simulink model "eBike_simulink_arduinoMega"  (R2021b)
settings: Solver=ode3  StartTime=0.0  StopTime=inf  FixedStep=0.1  RelTol=1e-3  EnableMultiTasking=on
libraries: arduinolib x17, simulink x9, dspsigops x1
settings Model: FPTRunName=Active  ExtModeTrigDuration=2  Creator=HP  LastModifiedBy=adhip
settings SolverCC: AlgebraicLoopSolver=TrustRegion
settings DataIOCC: LimitDataPoints=on  SaveFormat=Array
settings OptimizationCC: ExpressionDepthLimit=2147483647  LifeSpan=Inf  MaxStackSize=64
settings DebuggingCC: MergeDetectMultiDrivingBlocksExec=none  FcnCallInpInsideContextMsg=warning  AllowSymbolicDim=off  StateNameClashWarn=warning  SFUnexpectedBacktrackingDiag=warning  SFNoUnconditionalDefaultTransitionDiag=warning  SFExecutionAtInitializationDiag=none  SFMachineParentedDataDiag=warning  ArithmeticOperatorsInVariantConditions=warning
settings HardwareCC: ProdBitPerInt=16  ProdBitPerPointer=16  ProdBitPerSizeT=16  ProdBitPerPtrDiffT=16  ProdLargestAtomicFloat=None  ProdWordSize=8  ProdHWDeviceType=Atmel->AVR  UseEmbeddedCoderFeatures=off  UseSimulinkCoderFeatures=off
settings ModelReferenceCC: PropagateSignalLabelsOutOfModel=off
settings SFSimCC: SimUseLocalCustomCode=off  CustomCodeUndefinedFunction=UseInterfaceOnly
settings RTWCC: Description=Embedded Coder  SystemTargetFile=ert.tlc  HardwareBoard=Arduino Mega 2560  TemplateMakefile=ert_default_tmf  GenerateReport=on  RTWVerbose=off  RTWUseLocalCustomCode=off  Toolchain=Arduino AVR  BuildConfiguration=Faster Runs  LaunchReport=on
settings CodeAppCC: ForceParamTrailComments=on  OperatorAnnotations=on  MangleLength=10  StateflowObjectComments=on  MATLABSourceComments=on
settings ERTTargetCC: MultiwordLength=2048  ERTCustomFileBanners=off  SupportContinuousTime=on  SupportNonInlinedSFcns=on  RemoveResetFunc=off  ModelStepFunctionPrototypeControlCompliant=off
settings ConfigComp: CovMetricSettings=dw  CovSaveCumulativeToWorkspaceVar=on  CovSaveSingleToWorkspaceVar=on  CovExternalEMLEnable=off  CovSFcnEnable=off

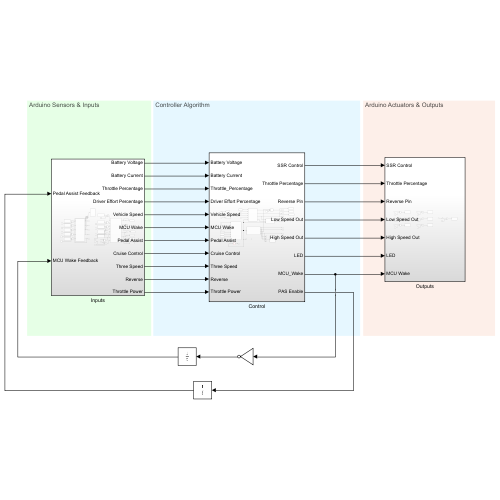
[thumbnail: Simulink's stored preview of the top-level diagram]
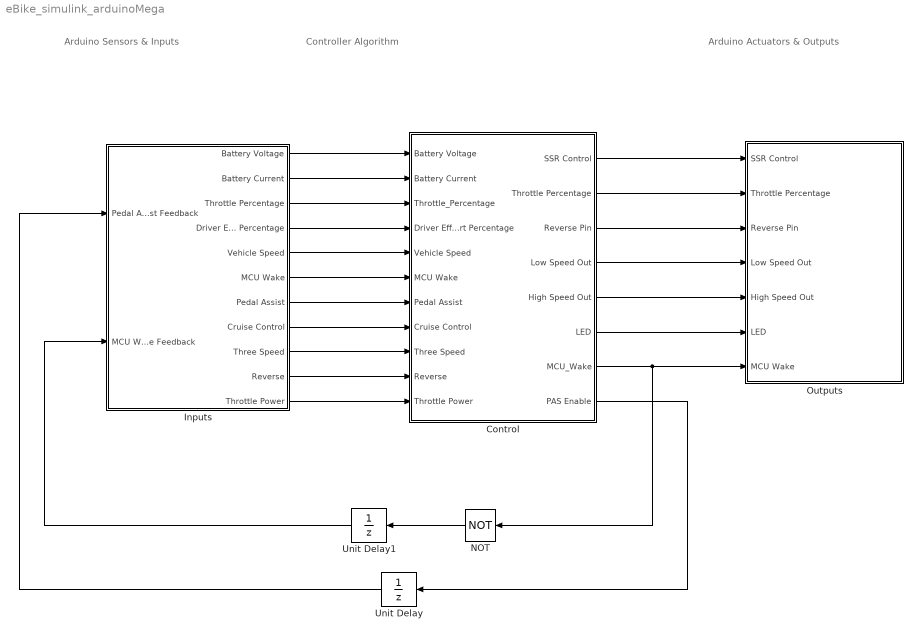
== system eBike_simulink_arduinoMega ==
  note: Arduino Actuators & Outputs
  note: Arduino Sensors & Inputs
  note: Controller Algorithm
  Control : Subsystem
  Inputs : Subsystem
  NOT : Logic  Operator=NOT  IconShape=distinctive  AllPortsSameDT=off  OutDataTypeStr=boolean
  Outputs : Subsystem
  Unit Delay : UnitDelay  SampleTime=-1  HasFrameUpgradeWarning=on
  Unit Delay1 : UnitDelay  SampleTime=-1  HasFrameUpgradeWarning=on
  wires:
  Inputs/1(Battery Voltage) -> Control/1(Battery Voltage)
  Inputs/2(Battery Current) -> Control/2(Battery Current)
  Inputs/3(Throttle Percentage) -> Control/3(Throttle_Percentage)
  Inputs/4(Driver Effort Percentage) -> Control/4(Driver Effort Percentage)
  Inputs/5(Vehicle Speed) -> Control/5(Vehicle Speed)
  Inputs/6(MCU Wake) -> Control/6(MCU Wake)
  Inputs/7(Pedal Assist) -> Control/7(Pedal Assist)
  Inputs/8(Cruise Control) -> Control/8(Cruise Control)
  Inputs/9(Three Speed) -> Control/9(Three Speed)
  Inputs/10(Reverse) -> Control/10(Reverse)
  Control/8(PAS Enable) -> Unit Delay/1
  Inputs/11(Throttle Power) -> Control/11(Throttle Power)
  Unit Delay/1 -> Inputs/1(Pedal Assist Feedback)
  Control/7(MCU_Wake) -> NOT/1, Outputs/7(MCU Wake)
  Unit Delay1/1 -> Inputs/2(MCU Wake Feedback)
  Control/1(SSR Control) -> Outputs/1(SSR Control)
  Control/3(Reverse Pin) -> Outputs/3(Reverse Pin)
  Control/4(Low Speed Out) -> Outputs/4(Low Speed Out)
  Control/5(High Speed Out) -> Outputs/5(High Speed Out)
  Control/6(LED) -> Outputs/6(LED)
  Control/2(Throttle Percentage) -> Outputs/2(Throttle Percentage)
  NOT/1 -> Unit Delay1/1

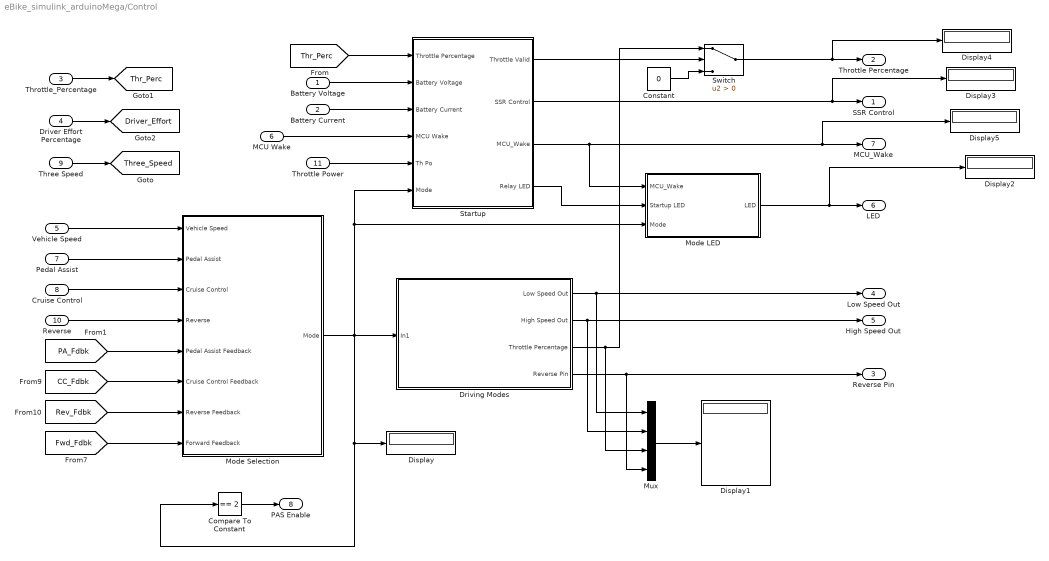
== system eBike_simulink_arduinoMega/Control ==
  Battery Voltage : Inport
  Battery Current : Inport  Port=2
  Throttle_Percentage : Inport  Port=3
  Driver Effort Percentage : Inport  Port=4
  Vehicle Speed : Inport  Port=5
  MCU Wake : Inport  Port=6
  Pedal Assist : Inport  Port=7
  Cruise Control : Inport  Port=8
  Three Speed : Inport  Port=9
  Reverse : Inport  Port=10
  Throttle Power : Inport  Port=11
  Compare To Constant : simulink/Logic and Bit Operations/Compare To Constant  relop===  const=2  OutDataTypeStr=boolean
  Constant : Constant  Value=0
  Display{,1..5} (6 alike) : Display
  Driving Modes : Subsystem
  Mode LED : Subsystem
  Mode Selection : Subsystem
  Mux : Mux
  Startup : Subsystem
  Switch : Switch  Criteria=u2 > Threshold
  SSR Control : Outport
  Throttle Percentage : Outport  Port=2
  Reverse Pin : Outport  Port=3
  Low Speed Out : Outport  Port=4
  High Speed Out : Outport  Port=5
  LED : Outport  Port=6
  MCU_Wake : Outport  Port=7
  PAS Enable : Outport  Port=8
  tag scope: Driver_Effort=global, Thr_Perc=global, Three_Speed=global
  wires:
  Pedal Assist/1 -> Mode Selection/2(Pedal Assist)
  Cruise Control/1 -> Mode Selection/3(Cruise Control)
  Reverse/1 -> Mode Selection/4(Reverse)
  Vehicle Speed/1 -> Mode Selection/1(Vehicle Speed)
  Three Speed/1 -> [Three_Speed]
  Throttle_Percentage/1 -> [Thr_Perc]
  Driver Effort Percentage/1 -> [Driver_Effort]
  [CC_Fdbk] -> Mode Selection/6(Cruise Control Feedback)
  [Fwd_Fdbk] -> Mode Selection/8(Forward Feedback)
  [Rev_Fdbk] -> Mode Selection/7(Reverse Feedback)
  Driving Modes/1(Low Speed Out) -> Mux/1, Low Speed Out/1
  Driving Modes/2(High Speed Out) -> Mux/2, High Speed Out/1
  Driving Modes/3(Throttle Percentage) -> Mux/3, Switch/1
  Driving Modes/4(Reverse Pin) -> Mux/4, Reverse Pin/1
  Battery Current/1 -> Startup/3(Battery Current)
  [Thr_Perc] -> Startup/1(Throttle Percentage)
  [PA_Fdbk] -> Mode Selection/5(Pedal Assist Feedback)
  Compare To Constant/1 -> PAS Enable/1
  Battery Voltage/1 -> Startup/2(Battery Voltage)
  Throttle Power/1 -> Startup/5(Th Po)
  Startup/4(Relay LED) -> Mode LED/2(Startup LED)
  Startup/3(MCU_Wake) -> Display5/1, MCU_Wake/1, Mode LED/1(MCU_Wake)
  Startup/1(Throttle Valid) -> Switch/2
  Constant/1 -> Switch/3
  Switch/1 -> Display4/1, Throttle Percentage/1
  Startup/2(SSR Control) -> Display3/1, SSR Control/1
  Mode LED/1(LED) -> Display2/1, LED/1
  Mode Selection/1(Mode) -> Display/1, Compare To Constant/1, Startup/6(Mode), Mode LED/3(Mode), Driving Modes/1(In1)
  Mux/1 -> Display1/1
  MCU Wake/1 -> Startup/4(MCU Wake)

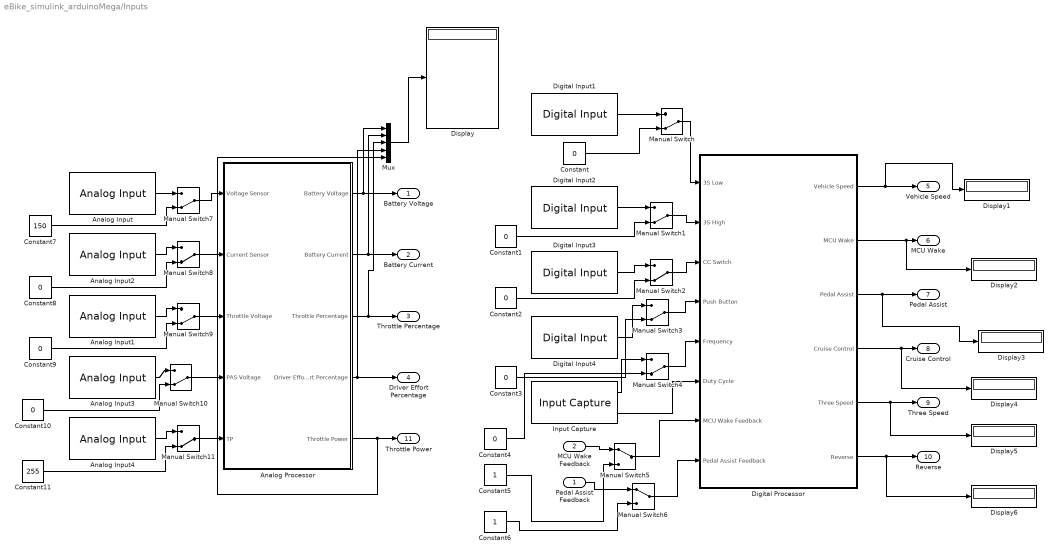
== system eBike_simulink_arduinoMega/Inputs ==
  Pedal Assist Feedback : Inport
  MCU Wake Feedback : Inport  Port=2
  Analog Input : arduinolib/Analog Input  pinNumber=15  ReadResultsOnly=off  ConversionTriggerSource=Software  ExternalTriggerType=uint32( 0 )  OutputDataType=uint16  EnableConversionCompleteNotify=off  EnableOuputStatus=off  SampleTime=-1  blockPlatform=arduino
  Analog Input1 : arduinolib/Analog Input  pinNumber=13  ReadResultsOnly=off  ConversionTriggerSource=Software  ExternalTriggerType=uint32( 0 )  OutputDataType=uint16  EnableConversionCompleteNotify=off  EnableOuputStatus=off  SampleTime=-1  blockPlatform=arduino
  Analog Input2 : arduinolib/Analog Input  pinNumber=14  ReadResultsOnly=off  ConversionTriggerSource=Software  ExternalTriggerType=uint32( 0 )  OutputDataType=uint16  EnableConversionCompleteNotify=off  EnableOuputStatus=off  SampleTime=-1  blockPlatform=arduino
  Analog Input3 : arduinolib/Analog Input  pinNumber=12  ReadResultsOnly=off  ConversionTriggerSource=Software  ExternalTriggerType=uint32( 0 )  OutputDataType=uint16  EnableConversionCompleteNotify=off  EnableOuputStatus=off  SampleTime=-1  blockPlatform=arduino
  Analog Input4 : arduinolib/Analog Input  pinNumber=11  ReadResultsOnly=off  ConversionTriggerSource=Software  ExternalTriggerType=uint32( 0 )  OutputDataType=uint16  EnableConversionCompleteNotify=off  EnableOuputStatus=off  SampleTime=-1  blockPlatform=arduino
  Analog Processor : Subsystem
  Constant{,1..4,8..10} (8 alike) : Constant  Value=0
  Constant11 : Constant  Value=255
  Constant5 : Constant
  Constant6 : Constant
  Constant7 : Constant  Value=150
  Digital Input1 : arduinolib/Digital Input  pinNumber=4  mode=Input Pullup  Direction=input  SampleTime=0.1  blockPlatform=arduino
  Digital Input2 : arduinolib/Digital Input  pinNumber=5  mode=Input Pullup  Direction=input  SampleTime=0.1  blockPlatform=arduino
  Digital Input3 : arduinolib/Digital Input  pinNumber=2  mode=Input Pullup  Direction=input  SampleTime=0.1  blockPlatform=arduino
  Digital Input4 : arduinolib/Digital Input  pinNumber=3  mode=Input Pullup  Direction=input  SampleTime=0.1  blockPlatform=arduino
  Digital Processor : Subsystem
  Display{,1..6} (7 alike) : Display
  Input Capture : arduinolib/Input Capture  InputCapturePinNumber=48  SampleTime=0.1
      settings: SourceProductBaseCode=ARDUINO
  Manual Switch{,1..4,7..11} (10 alike) : ManualSwitch  CurrentSetting=0
  Manual Switch5 : ManualSwitch
  Manual Switch6 : ManualSwitch
  Mux : Mux  Inputs=5
  Battery Voltage : Outport
  Battery Current : Outport  Port=2
  Throttle Percentage : Outport  Port=3
  Driver Effort Percentage : Outport  Port=4
  Vehicle Speed : Outport  Port=5
  MCU Wake : Outport  Port=6
  Pedal Assist : Outport  Port=7
  Cruise Control : Outport  Port=8
  Three Speed : Outport  Port=9
  Reverse : Outport  Port=10
  Throttle Power : Outport  Port=11
  wires:
  Manual Switch7/1 -> Analog Processor/1(Voltage Sensor)
  Manual Switch8/1 -> Analog Processor/2(Current Sensor)
  Manual Switch9/1 -> Analog Processor/3(Throttle Voltage)
  Manual Switch10/1 -> Analog Processor/4(PAS Voltage)
  Manual Switch/1 -> Digital Processor/1(3S Low)
  Manual Switch1/1 -> Digital Processor/2(3S High)
  Manual Switch2/1 -> Digital Processor/3(CC Switch)
  Manual Switch3/1 -> Digital Processor/4(Push Button)
  Manual Switch4/1 -> Digital Processor/5(Frequency)
  Input Capture/2 -> Digital Processor/6(Duty Cycle)
  Analog Processor/1(Battery Voltage) -> Mux/1, Battery Voltage/1
  Analog Processor/2(Battery Current) -> Mux/2, Battery Current/1
  Analog Processor/3(Throttle Percentage) -> Mux/3, Throttle Percentage/1
  Analog Processor/4(Driver Effort Percentage) -> Driver Effort Percentage/1, Mux/4
  Digital Processor/1(Vehicle Speed) -> Display1/1, Vehicle Speed/1
  Digital Processor/2(MCU Wake) -> Display2/1, MCU Wake/1
  Digital Processor/3(Pedal Assist) -> Display3/1, Pedal Assist/1
  Digital Processor/4(Cruise Control) -> Display4/1, Cruise Control/1
  Digital Processor/5(Three Speed) -> Display5/1, Three Speed/1
  Manual Switch6/1 -> Digital Processor/8(Pedal Assist Feedback)
  Manual Switch5/1 -> Digital Processor/7(MCU Wake Feedback)
  Analog Processor/5(Throttle Power) -> Mux/5, Throttle Power/1
  Manual Switch11/1 -> Analog Processor/5(TP)
  Digital Input1/1 -> Manual Switch/1
  Constant/1 -> Manual Switch/2
  Digital Input2/1 -> Manual Switch1/1
  Constant1/1 -> Manual Switch1/2
  Digital Input3/1 -> Manual Switch2/1
  Constant2/1 -> Manual Switch2/2
  Digital Input4/1 -> Manual Switch3/1
  Constant3/1 -> Manual Switch3/2
  Input Capture/1 -> Manual Switch4/1
  Constant4/1 -> Manual Switch4/2
  MCU Wake Feedback/1 -> Manual Switch5/1
  Constant5/1 -> Manual Switch5/2
  Pedal Assist Feedback/1 -> Manual Switch6/1
  Constant6/1 -> Manual Switch6/2
  Analog Input/1 -> Manual Switch7/1
  Constant7/1 -> Manual Switch7/2
  Analog Input2/1 -> Manual Switch8/1
  Constant8/1 -> Manual Switch8/2
  Analog Input1/1 -> Manual Switch9/1
  Constant9/1 -> Manual Switch9/2
  Analog Input3/1 -> Manual Switch10/1
  Constant10/1 -> Manual Switch10/2
  Analog Input4/1 -> Manual Switch11/1
  Constant11/1 -> Manual Switch11/2
  Mux/1 -> Display/1
  Digital Processor/6(Reverse) -> Display6/1, Reverse/1

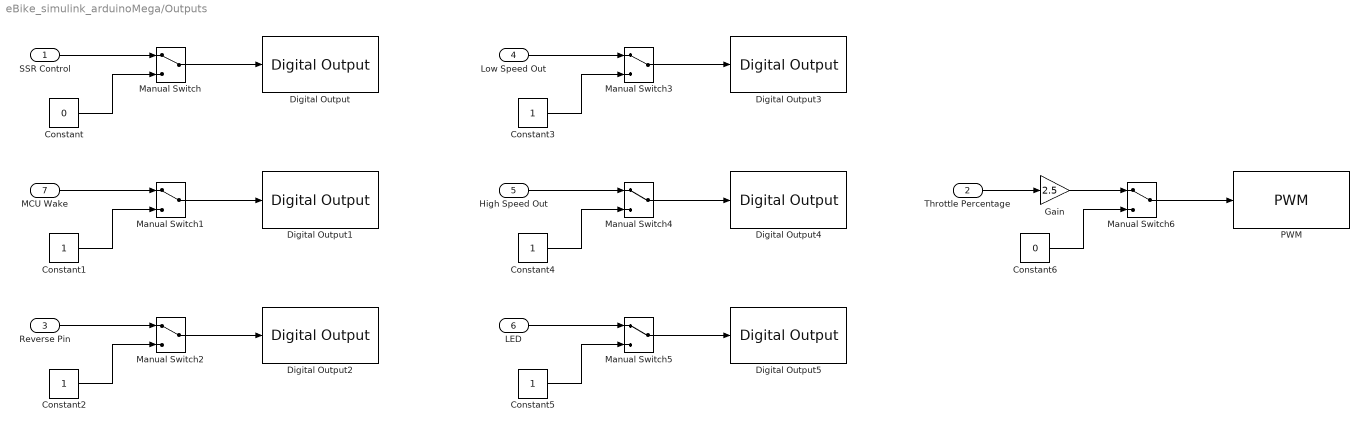
== system eBike_simulink_arduinoMega/Outputs ==
  SSR Control : Inport
  Throttle Percentage : Inport  Port=2
  Reverse Pin : Inport  Port=3
  Low Speed Out : Inport  Port=4
  High Speed Out : Inport  Port=5
  LED : Inport  Port=6
  MCU Wake : Inport  Port=7
  Constant : Constant  Value=0
  Constant{1..5} (5 alike) : Constant
  Constant6 : Constant  Value=0
  Digital Output : arduinolib/Digital Output  pinNumber=9  Direction=output  blockPlatform=arduino
  Digital Output1 : arduinolib/Digital Output  pinNumber=10  Direction=output  blockPlatform=arduino
  Digital Output2 : arduinolib/Digital Output  pinNumber=6  Direction=output  blockPlatform=arduino
  Digital Output3 : arduinolib/Digital Output  pinNumber=8  Direction=output  blockPlatform=arduino
  Digital Output4 : arduinolib/Digital Output  pinNumber=7  Direction=output  blockPlatform=arduino
  Digital Output5 : arduinolib/Digital Output  pinNumber=11  Direction=output  blockPlatform=arduino
  Gain : Gain  Gain=2.5
  Manual Switch{,1..6} (7 alike) : ManualSwitch
  PWM : arduinolib/PWM  pinNumber=12  frequencyType=Default  desiredFrequency=490.2  achievableFrequency=490.2
  wires:
  Manual Switch/1 -> Digital Output/1
  Constant/1 -> Manual Switch/2
  SSR Control/1 -> Manual Switch/1
  MCU Wake/1 -> Manual Switch1/1
  Constant1/1 -> Manual Switch1/2
  Manual Switch1/1 -> Digital Output1/1
  Manual Switch2/1 -> Digital Output2/1
  Constant2/1 -> Manual Switch2/2
  Reverse Pin/1 -> Manual Switch2/1
  LED/1 -> Manual Switch5/1
  Constant5/1 -> Manual Switch5/2
  Manual Switch5/1 -> Digital Output5/1
  Manual Switch4/1 -> Digital Output4/1
  Constant4/1 -> Manual Switch4/2
  High Speed Out/1 -> Manual Switch4/1
  Low Speed Out/1 -> Manual Switch3/1
  Constant3/1 -> Manual Switch3/2
  Manual Switch3/1 -> Digital Output3/1
  Manual Switch6/1 -> PWM/1
  Constant6/1 -> Manual Switch6/2
  Throttle Percentage/1 -> Gain/1
  Gain/1 -> Manual Switch6/1

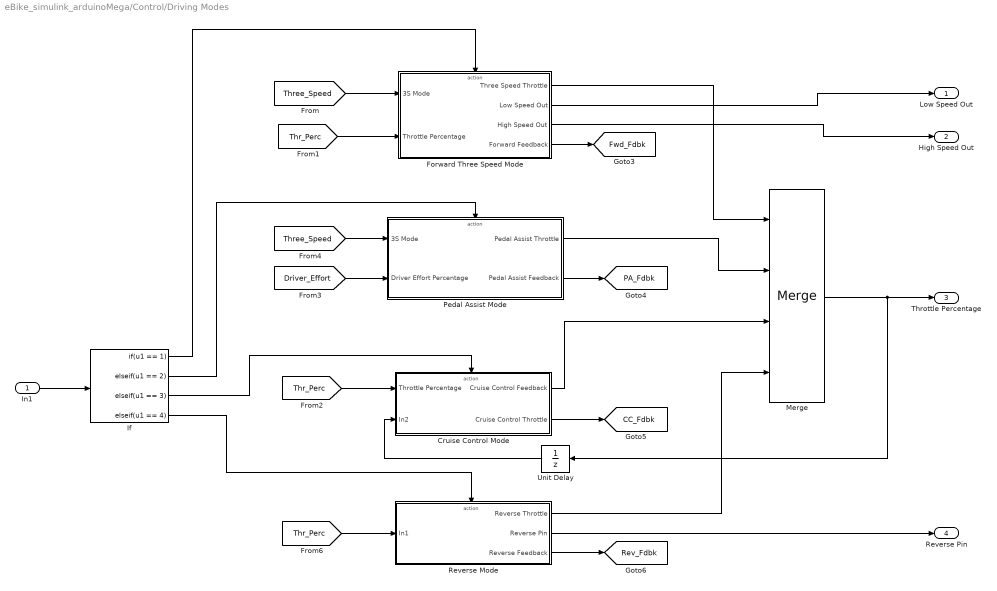
== system eBike_simulink_arduinoMega/Control/Driving Modes ==
  In1 : Inport
  Cruise Control Mode : Subsystem  TreatAsAtomicUnit=on
  Forward Three Speed Mode : Subsystem  TreatAsAtomicUnit=on
  If : If  IfExpression=u1 == 1  ElseIfExpressions=u1 == 2,u1 == 3,u1 == 4  ShowElse=off
  Merge : Merge  Inputs=4
  Pedal Assist Mode : Subsystem  TreatAsAtomicUnit=on
  Reverse Mode : Subsystem  TreatAsAtomicUnit=on
  Unit Delay : UnitDelay  SampleTime=-1  HasFrameUpgradeWarning=on
  Low Speed Out : Outport
  High Speed Out : Outport  Port=2
  Throttle Percentage : Outport  Port=3
  Reverse Pin : Outport  Port=4
  tag scope: CC_Fdbk=global, Fwd_Fdbk=global, PA_Fdbk=global, Rev_Fdbk=global
  wires:
  [Thr_Perc] -> Cruise Control Mode/1(Throttle Percentage)
  Reverse Mode/1(Reverse Throttle) -> Merge/4
  Cruise Control Mode/1(Cruise Control Feedback) -> Merge/3
  If/4 -> Reverse Mode/Action
  Reverse Mode/2(Reverse Pin) -> Reverse Pin/1
  [Thr_Perc] -> Reverse Mode/1(In1)
  Forward Three Speed Mode/1(Three Speed Throttle) -> Merge/1
  Pedal Assist Mode/1(Pedal Assist Throttle) -> Merge/2
  [Three_Speed] -> Forward Three Speed Mode/1(3S Mode)
  If/2 -> Pedal Assist Mode/Action
  If/3 -> Cruise Control Mode/Action
  Forward Three Speed Mode/3(High Speed Out) -> High Speed Out/1
  Reverse Mode/3(Reverse Feedback) -> [Rev_Fdbk]
  Forward Three Speed Mode/2(Low Speed Out) -> Low Speed Out/1
  If/1 -> Forward Three Speed Mode/Action
  In1/1 -> If/1
  Forward Three Speed Mode/4(Forward Feedback) -> [Fwd_Fdbk]
  [Driver_Effort] -> Pedal Assist Mode/2(Driver Effort Percentage)
  [Thr_Perc] -> Forward Three Speed Mode/2(Throttle Percentage)
  Cruise Control Mode/2(Cruise Control Throttle) -> [CC_Fdbk]
  [Three_Speed] -> Pedal Assist Mode/1(3S Mode)
  Pedal Assist Mode/2(Pedal Assist Feedback) -> [PA_Fdbk]
  Merge/1 -> Unit Delay/1, Throttle Percentage/1
  Unit Delay/1 -> Cruise Control Mode/2(In2)

== system eBike_simulink_arduinoMega/Control/Mode LED ==
  MCU_Wake : Inport
  Startup LED : Inport  Port=2
  Mode : Inport  Port=3
  Chart : Stateflow chart  TreatAsAtomicUnit=on
  Compare To Constant : simulink/Logic and Bit Operations/Compare To Constant  relop===  const=3.0  OutDataTypeStr=boolean
  Compare To Constant1 : simulink/Logic and Bit Operations/Compare To Constant  relop===  const=4  OutDataTypeStr=boolean
  Compare To Constant2 : simulink/Logic and Bit Operations/Compare To Constant  relop===  const=2  OutDataTypeStr=boolean
  Data Type Conversion : DataTypeConversion  OutDataTypeStr=boolean
  LED : Outport
  wires:
  Startup LED/1 -> Data Type Conversion/1
  Mode/1 -> Compare To Constant2/1, Compare To Constant1/1, Compare To Constant/1
  Compare To Constant/1 -> Chart/3(CC_LED)
  Compare To Constant1/1 -> Chart/4(Rev_LED)
  Compare To Constant2/1 -> Chart/5(PA_LED)
  MCU_Wake/1 -> Chart/1(MCU_Wake)
  Chart/1(relay_LED) -> LED/1
  Data Type Conversion/1 -> Chart/2(Startup_LED)

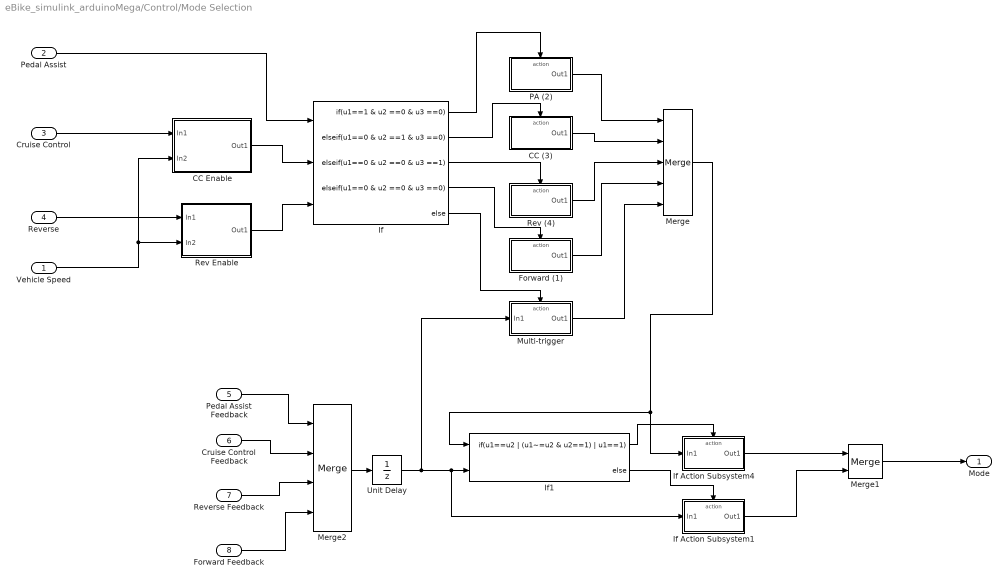
== system eBike_simulink_arduinoMega/Control/Mode Selection ==
  Vehicle Speed : Inport
  Pedal Assist : Inport  Port=2
  Cruise Control : Inport  Port=3
  Reverse : Inport  Port=4
  Pedal Assist Feedback : Inport  Port=5
  Cruise Control Feedback : Inport  Port=6
  Reverse Feedback : Inport  Port=7
  Forward Feedback : Inport  Port=8
  CC (3) : Subsystem  TreatAsAtomicUnit=on
  CC Enable : Subsystem
  Forward (1) : Subsystem  TreatAsAtomicUnit=on
  If : If  NumInputs=3  IfExpression=u1==1 & u2 ==0 & u3 ==0  ElseIfExpressions=u1==0 & u2 ==1 & u3 ==0,u1==0 & u2 ==0 & u3 ==1,u1==0 & u2 ==0 & u3 ==0
  If Action Subsystem1 : Subsystem  TreatAsAtomicUnit=on
  If Action Subsystem4 : Subsystem  TreatAsAtomicUnit=on
  If1 : If  NumInputs=2  IfExpression=u1==u2 | (u1~=u2 & u2==1) | u1==1
  Merge : Merge  Inputs=5
  Merge1 : Merge
  Merge2 : Merge  Inputs=4
  Multi-trigger : Subsystem  TreatAsAtomicUnit=on
  PA (2) : Subsystem  TreatAsAtomicUnit=on
  Rev (4) : Subsystem  TreatAsAtomicUnit=on
  Rev Enable : Subsystem
  Unit Delay : UnitDelay  InitialCondition=1  SampleTime=-1  HasFrameUpgradeWarning=on
  Mode : Outport
  wires:
  Pedal Assist/1 -> If/1
  If/1 -> PA (2)/Action
  If/2 -> CC (3)/Action
  If/3 -> Rev (4)/Action
  PA (2)/1(Out1) -> Merge/1
  CC (3)/1(Out1) -> Merge/2
  Rev (4)/1(Out1) -> Merge/3
  Forward (1)/1(Out1) -> Merge/4
  Pedal Assist Feedback/1 -> Merge2/1
  Cruise Control Feedback/1 -> Merge2/2
  Reverse Feedback/1 -> Merge2/3
  Forward Feedback/1 -> Merge2/4
  Merge2/1 -> Unit Delay/1
  Merge/1 -> If1/1, If Action Subsystem4/1(In1)
  If1/1 -> If Action Subsystem4/Action
  If Action Subsystem4/1(Out1) -> Merge1/1
  Merge1/1 -> Mode/1
  Vehicle Speed/1 -> Rev Enable/2(In2), CC Enable/2(In2)
  If1/2 -> If Action Subsystem1/Action
  If Action Subsystem1/1(Out1) -> Merge1/2
  If/4 -> Forward (1)/Action
  If/5 -> Multi-trigger/Action
  Reverse/1 -> Rev Enable/1(In1)
  Rev Enable/1(Out1) -> If/3
  Cruise Control/1 -> CC Enable/1(In1)
  CC Enable/1(Out1) -> If/2
  Multi-trigger/1(Out1) -> Merge/5
  Unit Delay/1 -> Multi-trigger/1(In1), If Action Subsystem1/1(In1), If1/2

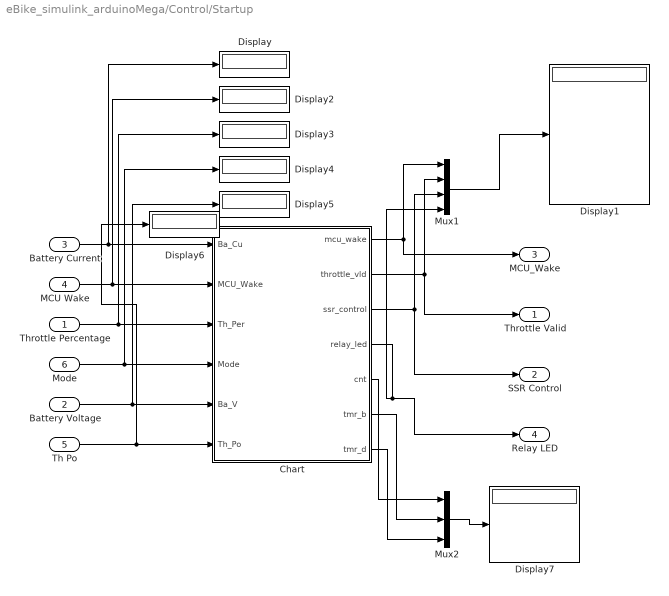
== system eBike_simulink_arduinoMega/Control/Startup ==
  Throttle Percentage : Inport
  Battery Voltage : Inport  Port=2
  Battery Current : Inport  Port=3
  MCU Wake : Inport  Port=4
  Th Po : Inport  Port=5
  Mode : Inport  Port=6
  Chart : Stateflow chart  TreatAsAtomicUnit=on
  Display{,1..7} (8 alike) : Display
  Mux1 : Mux
  Mux2 : Mux  Inputs=3
  Throttle Valid : Outport
  SSR Control : Outport  Port=2
  MCU_Wake : Outport  Port=3
  Relay LED : Outport  Port=4
  wires:
  MCU Wake/1 -> Display2/1, Chart/2(MCU_Wake)
  Throttle Percentage/1 -> Display3/1, Chart/3(Th_Per)
  Mode/1 -> Display4/1, Chart/4(Mode)
  Battery Voltage/1 -> Display5/1, Chart/5(Ba_V)
  Th Po/1 -> Display6/1, Chart/6(Th_Po)
  Chart/1(mcu_wake) -> MCU_Wake/1, Mux1/1
  Chart/2(throttle_vld) -> Throttle Valid/1, Mux1/2
  Chart/3(ssr_control) -> SSR Control/1, Mux1/3
  Chart/4(relay_led) -> Relay LED/1, Mux1/4
  Battery Current/1 -> Display/1, Chart/1(Ba_Cu)
  Mux1/1 -> Display1/1
  Chart/5(cnt) -> Mux2/1
  Chart/6(tmr_b) -> Mux2/2
  Chart/7(tmr_d) -> Mux2/3
  Mux2/1 -> Display7/1

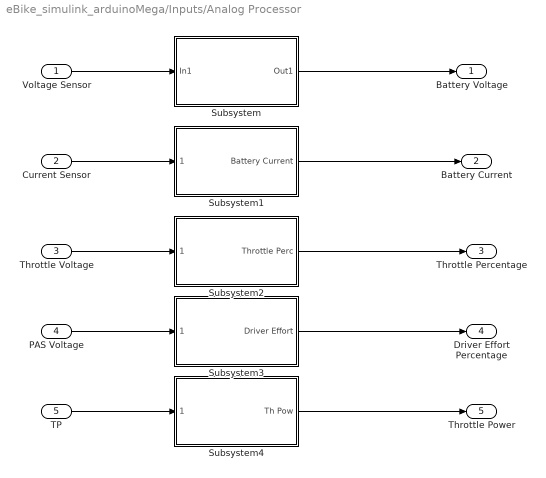
== system eBike_simulink_arduinoMega/Inputs/Analog Processor ==
  Voltage Sensor : Inport
  Current Sensor : Inport  Port=2
  Throttle Voltage : Inport  Port=3
  PAS Voltage : Inport  Port=4
  TP : Inport  Port=5
  Subsystem : Subsystem
  Subsystem1 : Subsystem
  Subsystem2 : Subsystem
  Subsystem3 : Subsystem
  Subsystem4 : Subsystem
  Battery Voltage : Outport
  Battery Current : Outport  Port=2
  Throttle Percentage : Outport  Port=3
  Driver Effort Percentage : Outport  Port=4
  Throttle Power : Outport  Port=5
  wires:
  Voltage Sensor/1 -> Subsystem/1(In1)
  Subsystem/1(Out1) -> Battery Voltage/1
  Current Sensor/1 -> Subsystem1/1(1)
  Subsystem1/1(Battery Current) -> Battery Current/1
  Throttle Voltage/1 -> Subsystem2/1(1)
  Subsystem2/1(Throttle Perc) -> Throttle Percentage/1
  PAS Voltage/1 -> Subsystem3/1(1)
  Subsystem3/1(Driver Effort) -> Driver Effort Percentage/1
  TP/1 -> Subsystem4/1(1)
  Subsystem4/1(Th Pow) -> Throttle Power/1

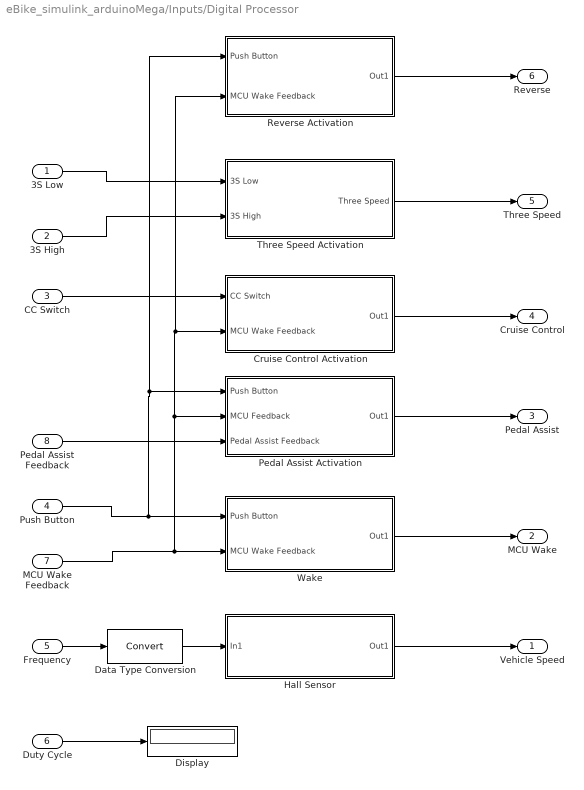
== system eBike_simulink_arduinoMega/Inputs/Digital Processor ==
  3S Low : Inport
  3S High : Inport  Port=2
  CC Switch : Inport  Port=3
  Push Button : Inport  Port=4
  Frequency : Inport  Port=5
  Duty Cycle : Inport  Port=6
  MCU Wake Feedback : Inport  Port=7
  Pedal Assist Feedback : Inport  Port=8
  Cruise Control Activation : Subsystem
  Data Type Conversion : DataTypeConversion
  Display : Display
  Hall Sensor : Subsystem
  Pedal Assist Activation : Subsystem
  Reverse Activation : Subsystem
  Three Speed Activation : Subsystem
  Wake : Subsystem
  Vehicle Speed : Outport
  MCU Wake : Outport  Port=2
  Pedal Assist : Outport  Port=3
  Cruise Control : Outport  Port=4
  Three Speed : Outport  Port=5
  Reverse : Outport  Port=6
  wires:
  Duty Cycle/1 -> Display/1
  Push Button/1 -> Reverse Activation/1(Push Button), Pedal Assist Activation/1(Push Button), Wake/1(Push Button)
  MCU Wake Feedback/1 -> Reverse Activation/2(MCU Wake Feedback), Cruise Control Activation/2(MCU Wake Feedback), Pedal Assist Activation/2(MCU Feedback), Wake/2(MCU Wake Feedback)
  Wake/1(Out1) -> MCU Wake/1
  Pedal Assist Activation/1(Out1) -> Pedal Assist/1
  CC Switch/1 -> Cruise Control Activation/1(CC Switch)
  Cruise Control Activation/1(Out1) -> Cruise Control/1
  3S Low/1 -> Three Speed Activation/1(3S Low)
  3S High/1 -> Three Speed Activation/2(3S High)
  Reverse Activation/1(Out1) -> Reverse/1
  Frequency/1 -> Data Type Conversion/1
  Hall Sensor/1(Out1) -> Vehicle Speed/1
  Three Speed Activation/1(Three Speed) -> Three Speed/1
  Pedal Assist Feedback/1 -> Pedal Assist Activation/3(Pedal Assist Feedback)
  Data Type Conversion/1 -> Hall Sensor/1(In1)

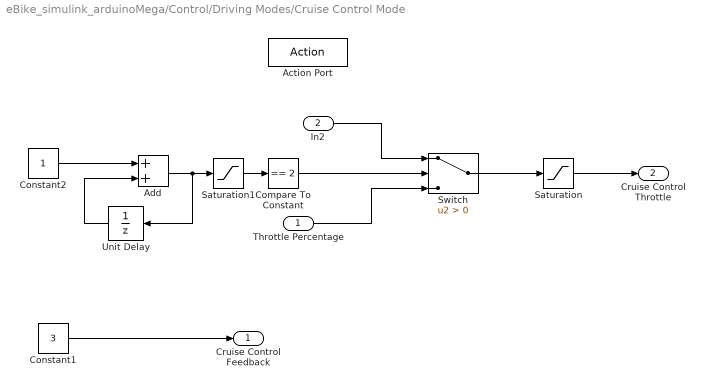
== system eBike_simulink_arduinoMega/Control/Driving Modes/Cruise Control Mode ==
  Throttle Percentage : Inport
  In2 : Inport  Port=2
  Action Port : ActionPort  InitializeStates=reset  ActionPortLabel=elseif(u1 == 3)
  Add : Sum
  Compare To Constant : simulink/Logic and Bit Operations/Compare To Constant  relop===  const=2  OutDataTypeStr=boolean
  Constant1 : Constant  Value=3
  Constant2 : Constant
  Saturation : Saturate  UpperLimit=50  LowerLimit=20
  Saturation1 : Saturate  UpperLimit=2  LowerLimit=0
  Switch : Switch  Criteria=u2 > Threshold
  Unit Delay : UnitDelay  SampleTime=-1  HasFrameUpgradeWarning=on
  Cruise Control Feedback : Outport
  Cruise Control Throttle : Outport  Port=2
  wires:
  In2/1 -> Switch/1
  Throttle Percentage/1 -> Switch/3
  Unit Delay/1 -> Add/2
  Saturation/1 -> Cruise Control Throttle/1
  Compare To Constant/1 -> Switch/2
  Constant1/1 -> Cruise Control Feedback/1
  Saturation1/1 -> Compare To Constant/1
  Add/1 -> Saturation1/1, Unit Delay/1
  Constant2/1 -> Add/1
  Switch/1 -> Saturation/1

== system eBike_simulink_arduinoMega/Control/Driving Modes/Forward Three Speed Mode ==
  3S Mode : Inport
  Throttle Percentage : Inport  Port=2
  Action Port : ActionPort  InitializeStates=reset  ActionPortLabel=if(u1 == 1)
  Constant : Constant
  High Speed Mapping : Subsystem  TreatAsAtomicUnit=on
  If : If  IfExpression=u1 == 1  ElseIfExpressions=u1 == 3
  Linear Mapping : Subsystem  TreatAsAtomicUnit=on
  Low Speed Mapping : Subsystem  TreatAsAtomicUnit=on
  Merge : Merge  Inputs=3
  Three Speed Throttle : Outport
  Low Speed Out : Outport  Port=2
  High Speed Out : Outport  Port=3
  Forward Feedback : Outport  Port=4  InitialOutput=1
  wires:
  3S Mode/1 -> If/1
  If/1 -> Low Speed Mapping/Action
  Throttle Percentage/1 -> Low Speed Mapping/1(Throttle Percentage), Linear Mapping/1(Throttle Percentage), High Speed Mapping/1(Throttle Percentage)
  Low Speed Mapping/1(Out1) -> Merge/1
  Linear Mapping/1(Out1) -> Merge/2
  High Speed Mapping/1(Out1) -> Merge/3
  Merge/1 -> Three Speed Throttle/1
  Low Speed Mapping/2(Low Speed Out) -> Low Speed Out/1
  High Speed Mapping/2(High Speed Out) -> High Speed Out/1
  Constant/1 -> Forward Feedback/1
  If/2 -> High Speed Mapping/Action
  If/3 -> Linear Mapping/Action

== system eBike_simulink_arduinoMega/Control/Driving Modes/Pedal Assist Mode ==
  3S Mode : Inport
  Driver Effort Percentage : Inport  Port=2
  Action Port : ActionPort  InitializeStates=reset  ActionPortLabel=elseif(u1 == 2)
  Constant : Constant  Value=2
  If : If  IfExpression=u1 == 1  ElseIfExpressions=u1 == 2,u1 == 3  ShowElse=off
  Level 1 : Subsystem  TreatAsAtomicUnit=on
  Level 2 : Subsystem  TreatAsAtomicUnit=on
  Level 3 : Subsystem  TreatAsAtomicUnit=on
  Merge : Merge  Inputs=3
  Pedal Assist Throttle : Outport
  Pedal Assist Feedback : Outport  Port=2
  wires:
  Constant/1 -> Pedal Assist Feedback/1
  Merge/1 -> Pedal Assist Throttle/1
  Level 3/1(L3 Throttle) -> Merge/3
  Level 2/1(L2 Throttle) -> Merge/2
  Level 1/1(L1 Throttle) -> Merge/1
  Driver Effort Percentage/1 -> Level 3/1(Driver Effort), Level 1/1(Driver Effort), Level 2/1(Driver Effort)
  If/3 -> Level 3/Action
  If/2 -> Level 2/Action
  If/1 -> Level 1/Action
  3S Mode/1 -> If/1

== system eBike_simulink_arduinoMega/Control/Driving Modes/Reverse Mode ==
  In1 : Inport
  Action Port : ActionPort  InitializeStates=reset  ActionPortLabel=elseif(u1 == 4)
  Constant1 : Constant
  Constant2 : Constant  Value=4
  Reverse Throttle : Outport
  Reverse Pin : Outport  Port=2  OutputWhenDisabled=reset  InitialOutput=0
  Reverse Feedback : Outport  Port=3
  wires:
  In1/1 -> Reverse Throttle/1
  Constant1/1 -> Reverse Pin/1
  Constant2/1 -> Reverse Feedback/1

== system eBike_simulink_arduinoMega/Control/Mode Selection/CC (3) ==
  Action Port : ActionPort  ActionPortLabel=elseif(u1==0 & u2 ==1 & u3 ==0)
  Constant : Constant  Value=3
  Out1 : Outport
  wires:
  Constant/1 -> Out1/1

== system eBike_simulink_arduinoMega/Control/Mode Selection/CC Enable ==
  In1 : Inport
  In2 : Inport  Port=2
  AND1 : Logic  IconShape=distinctive  AllPortsSameDT=off  OutDataTypeStr=boolean
  Constant1 : Constant  Value=10
  Less Than1 : RelationalOperator  Operator=<  OutDataTypeStr=boolean  RndMeth=Simplest
  Out1 : Outport
  wires:
  Constant1/1 -> Less Than1/2
  In1/1 -> AND1/1
  In2/1 -> Less Than1/1
  Less Than1/1 -> AND1/2
  AND1/1 -> Out1/1

== system eBike_simulink_arduinoMega/Control/Mode Selection/Forward (1) ==
  Action Port : ActionPort  ActionPortLabel=elseif(u1==0 & u2 ==0 & u3 ==0)
  Constant : Constant
  Out1 : Outport
  wires:
  Constant/1 -> Out1/1

== system eBike_simulink_arduinoMega/Control/Mode Selection/If Action Subsystem1 ==
  In1 : Inport
  Action Port : ActionPort  ActionPortLabel=else
  Out1 : Outport
  wires:
  In1/1 -> Out1/1

== system eBike_simulink_arduinoMega/Control/Mode Selection/If Action Subsystem4 ==
  In1 : Inport
  Action Port : ActionPort  ActionPortLabel=if(u1==u2 | (u1~=u2 & u2==1) | u1==1)
  Out1 : Outport
  wires:
  In1/1 -> Out1/1

== system eBike_simulink_arduinoMega/Control/Mode Selection/Multi-trigger ==
  In1 : Inport
  Action Port : ActionPort  ActionPortLabel=else
  Out1 : Outport
  wires:
  In1/1 -> Out1/1

== system eBike_simulink_arduinoMega/Control/Mode Selection/PA (2) ==
  Action Port : ActionPort  ActionPortLabel=if(u1==1 & u2 ==0 & u3 ==0)
  Constant : Constant  Value=2
  Out1 : Outport
  wires:
  Constant/1 -> Out1/1

== system eBike_simulink_arduinoMega/Control/Mode Selection/Rev (4) ==
  Action Port : ActionPort  ActionPortLabel=elseif(u1==0 & u2 ==0 & u3 ==1)
  Constant : Constant  Value=4
  Out1 : Outport
  wires:
  Constant/1 -> Out1/1

== system eBike_simulink_arduinoMega/Control/Mode Selection/Rev Enable ==
  In1 : Inport
  In2 : Inport  Port=2
  AND : Logic  IconShape=distinctive  AllPortsSameDT=off  OutDataTypeStr=boolean
  Constant : Constant
  Less Than : RelationalOperator  Operator=<  OutDataTypeStr=boolean  RndMeth=Simplest
  Out1 : Outport
  wires:
  AND/1 -> Out1/1
  In2/1 -> Less Than/1
  Constant/1 -> Less Than/2
  Less Than/1 -> AND/2
  In1/1 -> AND/1

== system eBike_simulink_arduinoMega/Inputs/Analog Processor/Subsystem ==
  In1 : Inport
  Add : Sum  Inputs=+-
  Add1 : Sum  Inputs=+-
  Divide : Product  Inputs=/*
  Gain : Gain  Gain=40
  High ADC Voltage Count : Constant  Value=255
  Low ADC Voltage Count : Constant  Value=0
  Out1 : Outport
  wires:
  In1/1 -> Add/1
  Low ADC Voltage Count/1 -> Add1/2, Add/2
  High ADC Voltage Count/1 -> Add1/1
  Add/1 -> Divide/2
  Add1/1 -> Divide/1
  Divide/1 -> Gain/1
  Gain/1 -> Out1/1

== system eBike_simulink_arduinoMega/Inputs/Analog Processor/Subsystem1 ==
  1 : Inport
  Add : Sum  Inputs=+-
  Add1 : Sum  Inputs=+-
  Divide : Product  Inputs=/*
  Gain : Gain  Gain=20
  High ADC Voltage Count : Constant  Value=255
  Low ADC Voltage Count : Constant  Value=0
  Battery Current : Outport
  wires:
  Gain/1 -> Battery Current/1
  Divide/1 -> Gain/1
  Add1/1 -> Divide/1
  Add/1 -> Divide/2
  High ADC Voltage Count/1 -> Add1/1
  Low ADC Voltage Count/1 -> Add/2, Add1/2
  1/1 -> Add/1

== system eBike_simulink_arduinoMega/Inputs/Analog Processor/Subsystem2 ==
  1 : Inport
  Add : Sum  Inputs=+-
  Add1 : Sum  Inputs=+-
  Divide : Product  Inputs=/*
  Gain : Gain  Gain=100
  High ADC Voltage Count : Constant  Value=255
  Low ADC Voltage Count : Constant  Value=0
  Throttle Perc : Outport
  wires:
  1/1 -> Add/1
  Low ADC Voltage Count/1 -> Add1/2, Add/2
  High ADC Voltage Count/1 -> Add1/1
  Add/1 -> Divide/2
  Add1/1 -> Divide/1
  Divide/1 -> Gain/1
  Gain/1 -> Throttle Perc/1

== system eBike_simulink_arduinoMega/Inputs/Analog Processor/Subsystem3 ==
  1 : Inport
  Add : Sum  Inputs=+-
  Add1 : Sum  Inputs=+-
  Divide : Product  Inputs=/*
  Gain : Gain  Gain=100
  High ADC Voltage Count : Constant  Value=255
  Low ADC Voltage Count : Constant  Value=0
  Driver Effort : Outport
  wires:
  Gain/1 -> Driver Effort/1
  Divide/1 -> Gain/1
  Add1/1 -> Divide/1
  Add/1 -> Divide/2
  High ADC Voltage Count/1 -> Add1/1
  Low ADC Voltage Count/1 -> Add/2, Add1/2
  1/1 -> Add/1

== system eBike_simulink_arduinoMega/Inputs/Analog Processor/Subsystem4 ==
  1 : Inport
  Add : Sum  Inputs=+-
  Add1 : Sum  Inputs=+-
  Divide : Product  Inputs=/*
  Gain : Gain  Gain=5
  "High ADC " : Constant  Value=255
  "Low ADC " : Constant  Value=0
  Th Pow : Outport
  wires:
  1/1 -> Add/1
  "Low ADC "/1 -> Add1/2, Add/2
  "High ADC "/1 -> Add1/1
  Add/1 -> Divide/2
  Add1/1 -> Divide/1
  Divide/1 -> Gain/1
  Gain/1 -> Th Pow/1

== system eBike_simulink_arduinoMega/Inputs/Digital Processor/Cruise Control Activation ==
  CC Switch : Inport
  MCU Wake Feedback : Inport  Port=2
  AND : Logic  IconShape=distinctive  AllPortsSameDT=off  OutDataTypeStr=boolean
  Constant : Constant
  Constant1 : Constant  Value=0
  Multiport Switch1 : MultiPortSwitch  DataPortOrder=Zero-based contiguous  Inputs=2  zeroidx=on
  Multiport Switch2 : MultiPortSwitch  DataPortOrder=Zero-based contiguous  Inputs=2  zeroidx=on
  NAND : Logic  Operator=NAND  IconShape=distinctive  AllPortsSameDT=off  OutDataTypeStr=boolean
  Unit Delay : UnitDelay  SampleTime=-1  HasFrameUpgradeWarning=on
  Out1 : Outport
  wires:
  Constant/1 -> Multiport Switch1/3
  AND/1 -> Multiport Switch1/1
  Multiport Switch2/1 -> Out1/1, Unit Delay/1
  Unit Delay/1 -> Multiport Switch1/2
  Multiport Switch1/1 -> Multiport Switch2/2
  Constant1/1 -> Multiport Switch2/3
  NAND/1 -> Multiport Switch2/1
  CC Switch/1 -> NAND/1, AND/1
  MCU Wake Feedback/1 -> NAND/2, AND/2

== system eBike_simulink_arduinoMega/Inputs/Digital Processor/Hall Sensor ==
  In1 : Inport
  Gain : Gain  Gain=2*pi
  Gain1 : Gain  Gain=18/5
  Pole Pairs : Gain  Gain=1/5
  Wheel radius : Gain  Gain=0.2
  Out1 : Outport
  wires:
  Wheel radius/1 -> Gain1/1
  Pole Pairs/1 -> Gain/1  "Mechanical Frequency"
  Gain/1 -> Wheel radius/1
  Gain1/1 -> Out1/1
  In1/1 -> Pole Pairs/1

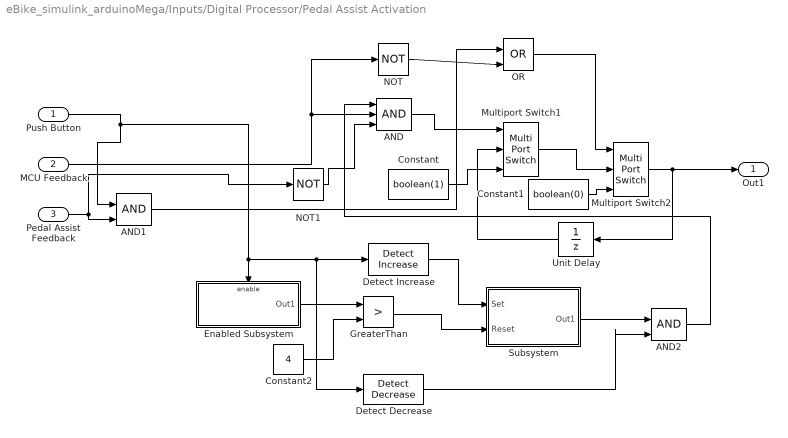
== system eBike_simulink_arduinoMega/Inputs/Digital Processor/Pedal Assist Activation ==
  Push Button : Inport
  MCU Feedback : Inport  Port=2
  Pedal Assist Feedback : Inport  Port=3
  AND : Logic  Inputs=3  IconShape=distinctive  AllPortsSameDT=off  OutDataTypeStr=boolean
  AND1 : Logic  IconShape=distinctive  AllPortsSameDT=off  OutDataTypeStr=boolean
  AND2 : Logic  IconShape=distinctive  AllPortsSameDT=off  OutDataTypeStr=boolean
  Constant : Constant  Value=boolean(1)
  Constant1 : Constant  Value=boolean(0)
  Constant2 : Constant  Value=4
  Detect Decrease : simulink/Logic and Bit Operations/Detect Decrease  vinit=0.0  OutDataTypeStr=boolean
  Detect Increase : simulink/Logic and Bit Operations/Detect Increase  vinit=0.0  OutDataTypeStr=boolean
  Enabled Subsystem : Subsystem  TreatAsAtomicUnit=on
  GreaterThan : RelationalOperator  Operator=>  OutDataTypeStr=boolean  RndMeth=Simplest
  Multiport Switch1 : MultiPortSwitch  DataPortOrder=Zero-based contiguous  Inputs=2  zeroidx=on
  Multiport Switch2 : MultiPortSwitch  DataPortOrder=Zero-based contiguous  Inputs=2  zeroidx=on
  NOT : Logic  Operator=NOT  IconShape=distinctive  AllPortsSameDT=off  OutDataTypeStr=boolean
  NOT1 : Logic  Operator=NOT  IconShape=distinctive  AllPortsSameDT=off  OutDataTypeStr=boolean
  OR : Logic  Operator=OR  IconShape=distinctive  AllPortsSameDT=off  OutDataTypeStr=boolean
  Subsystem : Subsystem
  Unit Delay : UnitDelay  SampleTime=-1  HasFrameUpgradeWarning=on
  Out1 : Outport
  wires:
  Push Button/1 -> AND1/1, Detect Decrease/1, Detect Increase/1, Enabled Subsystem/Enable
  AND/1 -> Multiport Switch1/1
  Constant/1 -> Multiport Switch1/3
  Constant1/1 -> Multiport Switch2/3
  Multiport Switch2/1 -> Unit Delay/1, Out1/1
  OR/1 -> Multiport Switch2/1
  Multiport Switch1/1 -> Multiport Switch2/2
  Unit Delay/1 -> Multiport Switch1/2
  MCU Feedback/1 -> NOT/1, AND/2
  Pedal Assist Feedback/1 -> NOT1/1, AND1/2
  AND1/1 -> OR/1
  NOT/1 -> OR/2
  NOT1/1 -> AND/3
  Detect Increase/1 -> Subsystem/1(Set)
  Constant2/1 -> GreaterThan/2
  GreaterThan/1 -> Subsystem/2(Reset)
  Enabled Subsystem/1(Out1) -> GreaterThan/1
  Detect Decrease/1 -> AND2/2
  Subsystem/1(Out1) -> AND2/1
  AND2/1 -> AND/1

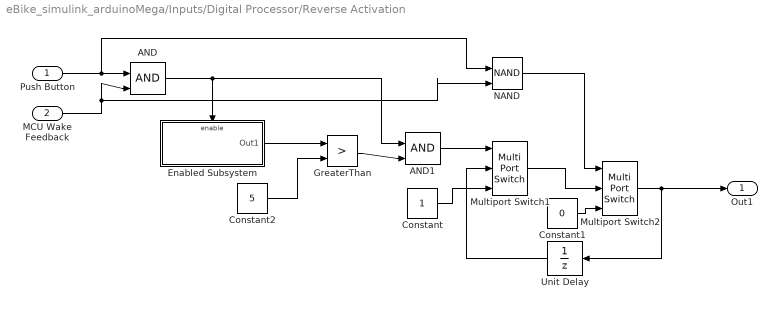
== system eBike_simulink_arduinoMega/Inputs/Digital Processor/Reverse Activation ==
  Push Button : Inport
  MCU Wake Feedback : Inport  Port=2
  AND : Logic  IconShape=distinctive  AllPortsSameDT=off  OutDataTypeStr=boolean
  AND1 : Logic  IconShape=distinctive  AllPortsSameDT=off  OutDataTypeStr=boolean
  Constant : Constant
  Constant1 : Constant  Value=0
  Constant2 : Constant  Value=5
  Enabled Subsystem : Subsystem  TreatAsAtomicUnit=on
  GreaterThan : RelationalOperator  Operator=>  OutDataTypeStr=boolean  RndMeth=Simplest
  Multiport Switch1 : MultiPortSwitch  DataPortOrder=Zero-based contiguous  Inputs=2  zeroidx=on
  Multiport Switch2 : MultiPortSwitch  DataPortOrder=Zero-based contiguous  Inputs=2  zeroidx=on
  NAND : Logic  Operator=NAND  IconShape=distinctive  AllPortsSameDT=off  OutDataTypeStr=boolean
  Unit Delay : UnitDelay  SampleTime=-1  HasFrameUpgradeWarning=on
  Out1 : Outport
  wires:
  Constant/1 -> Multiport Switch1/3
  Multiport Switch2/1 -> Out1/1, Unit Delay/1
  Unit Delay/1 -> Multiport Switch1/2
  Multiport Switch1/1 -> Multiport Switch2/2
  Constant1/1 -> Multiport Switch2/3
  NAND/1 -> Multiport Switch2/1
  AND/1 -> AND1/1, Enabled Subsystem/Enable
  Push Button/1 -> NAND/1, AND/1
  MCU Wake Feedback/1 -> NAND/2, AND/2
  Enabled Subsystem/1(Out1) -> GreaterThan/1
  Constant2/1 -> GreaterThan/2
  GreaterThan/1 -> AND1/2
  AND1/1 -> Multiport Switch1/1

== system eBike_simulink_arduinoMega/Inputs/Digital Processor/Three Speed Activation ==
  3S Low : Inport
  3S High : Inport  Port=2
  Add : Sum
  Gain : Gain
  Gain1 : Gain  Gain=2
  High : Constant  Value=3
  Low : Constant
  Medium : Constant  Value=2
  Multiport Switch : MultiPortSwitch
  Three Speed : Outport
  wires:
  3S Low/1 -> Gain/1
  3S High/1 -> Gain1/1
  Gain/1 -> Add/1
  Gain1/1 -> Add/2
  Add/1 -> Multiport Switch/1
  Low/1 -> Multiport Switch/2
  High/1 -> Multiport Switch/3
  Medium/1 -> Multiport Switch/4
  Multiport Switch/1 -> Three Speed/1

== system eBike_simulink_arduinoMega/Inputs/Digital Processor/Wake ==
  Push Button : Inport
  MCU Wake Feedback : Inport  Port=2
  AND : Logic  IconShape=distinctive  AllPortsSameDT=off  OutDataTypeStr=boolean
  AND2 : Logic  IconShape=distinctive  AllPortsSameDT=off  OutDataTypeStr=boolean
  Constant2 : Constant  Value=4
  Detect Decrease : simulink/Logic and Bit Operations/Detect Decrease  vinit=0.0  OutDataTypeStr=boolean
  Detect Increase : simulink/Logic and Bit Operations/Detect Increase  vinit=0.0  OutDataTypeStr=boolean
  Enabled Subsystem : Subsystem  TreatAsAtomicUnit=on
  GreaterThan : RelationalOperator  Operator=>  OutDataTypeStr=boolean  RndMeth=Simplest
  NOT : Logic  Operator=NOT  IconShape=distinctive  AllPortsSameDT=off  OutDataTypeStr=boolean
  Sample and Hold : dspsigops/Sample and Hold  trig=Rising edge  initCond=0  latchinput=off
  Subsystem : Subsystem
  Out1 : Outport
  wires:
  MCU Wake Feedback/1 -> NOT/1
  NOT/1 -> AND/2
  AND/1 -> Sample and Hold/Trigger, Sample and Hold/1
  Sample and Hold/1 -> Out1/1
  AND2/1 -> AND/1
  Subsystem/1(Out1) -> AND2/1
  Detect Decrease/1 -> AND2/2
  GreaterThan/1 -> Subsystem/2(Reset)
  Constant2/1 -> GreaterThan/2
  Detect Increase/1 -> Subsystem/1(Set)
  Enabled Subsystem/1(Out1) -> GreaterThan/1
  Push Button/1 -> Detect Decrease/1, Detect Increase/1, Enabled Subsystem/Enable

== system eBike_simulink_arduinoMega/Control/Driving Modes/Forward Three Speed Mode/High Speed Mapping ==
  Throttle Percentage : Inport
  Action Port : ActionPort  InitializeStates=reset  ActionPortLabel=elseif(u1 == 3)
  1-D Lookup Table : Lookup_n-D  NumberOfTableDimensions=1  BreakpointsForDimension1=[0:10:100]  Table=[0, 10, 20, 30, 40, 60, 80, 100, 100, 100, 100]  InternalRulePriority=Speed  RndMeth=Simplest  InputSameDT=on
  Constant : Constant
  Out1 : Outport
  High Speed Out : Outport  Port=2  OutputWhenDisabled=reset  InitialOutput=0
  wires:
  Throttle Percentage/1 -> 1-D Lookup Table/1
  1-D Lookup Table/1 -> Out1/1
  Constant/1 -> High Speed Out/1

== system eBike_simulink_arduinoMega/Control/Driving Modes/Forward Three Speed Mode/Linear Mapping ==
  Throttle Percentage : Inport
  Action Port : ActionPort  ActionPortLabel=else
  Out1 : Outport
  wires:
  Throttle Percentage/1 -> Out1/1

== system eBike_simulink_arduinoMega/Control/Driving Modes/Forward Three Speed Mode/Low Speed Mapping ==
  Throttle Percentage : Inport
  Action Port : ActionPort  InitializeStates=reset  ActionPortLabel=if(u1 == 1)
  1-D Lookup Table : Lookup_n-D  NumberOfTableDimensions=1  BreakpointsForDimension1=[0:10:100]  Table=[0:5:50]  InternalRulePriority=Speed  RndMeth=Simplest  InputSameDT=on
  Constant : Constant
  Out1 : Outport
  Low Speed Out : Outport  Port=2  OutputWhenDisabled=reset  InitialOutput=0
  wires:
  Throttle Percentage/1 -> 1-D Lookup Table/1
  1-D Lookup Table/1 -> Out1/1
  Constant/1 -> Low Speed Out/1

== system eBike_simulink_arduinoMega/Control/Driving Modes/Pedal Assist Mode/Level 1 ==
  Driver Effort : Inport
  Action Port : ActionPort  InitializeStates=reset  ActionPortLabel=if(u1 == 1)
  Gain : Gain  Gain=0.4
  Saturation : Saturate  UpperLimit=40  LowerLimit=10
  L1 Throttle : Outport
  wires:
  Driver Effort/1 -> Gain/1
  Gain/1 -> Saturation/1
  Saturation/1 -> L1 Throttle/1

== system eBike_simulink_arduinoMega/Control/Driving Modes/Pedal Assist Mode/Level 2 ==
  Driver Effort : Inport
  Action Port : ActionPort  InitializeStates=reset  ActionPortLabel=elseif(u1 == 2)
  Gain : Gain  Gain=0.7
  Saturation : Saturate  UpperLimit=70  LowerLimit=40
  L2 Throttle : Outport
  wires:
  Gain/1 -> Saturation/1
  Driver Effort/1 -> Gain/1
  Saturation/1 -> L2 Throttle/1

== system eBike_simulink_arduinoMega/Control/Driving Modes/Pedal Assist Mode/Level 3 ==
  Driver Effort : Inport
  Action Port : ActionPort  InitializeStates=reset  ActionPortLabel=elseif(u1 == 3)
  Gain : Gain
  Saturation : Saturate  UpperLimit=100  LowerLimit=70
  L3 Throttle : Outport
  wires:
  Saturation/1 -> L3 Throttle/1
  Gain/1 -> Saturation/1
  Driver Effort/1 -> Gain/1

== system eBike_simulink_arduinoMega/Inputs/Digital Processor/Pedal Assist Activation/Enabled Subsystem ==
  Enable : EnablePort  StatesWhenEnabling=reset
  Add : Sum
  Constant : Constant
  Unit Delay : UnitDelay  SampleTime=-1  HasFrameUpgradeWarning=on
  Out1 : Outport
  wires:
  Unit Delay/1 -> Add/2
  Constant/1 -> Add/1
  Add/1 -> Unit Delay/1, Out1/1

== system eBike_simulink_arduinoMega/Inputs/Digital Processor/Pedal Assist Activation/Subsystem ==
  Set : Inport
  Reset : Inport  Port=2
  Constant2 : Constant
  Constant3 : Constant  Value=0
  Multiport Switch3 : MultiPortSwitch  DataPortOrder=Zero-based contiguous  Inputs=2  zeroidx=on
  Multiport Switch4 : MultiPortSwitch  DataPortOrder=Zero-based contiguous  Inputs=2  zeroidx=on
  Unit Delay1 : UnitDelay  SampleTime=-1  HasFrameUpgradeWarning=on
  Out1 : Outport
  wires:
  Set/1 -> Multiport Switch3/1
  Constant2/1 -> Multiport Switch3/3
  Multiport Switch3/1 -> Multiport Switch4/2
  Unit Delay1/1 -> Multiport Switch3/2
  Multiport Switch4/1 -> Out1/1, Unit Delay1/1
  Constant3/1 -> Multiport Switch4/3
  Reset/1 -> Multiport Switch4/1

== system eBike_simulink_arduinoMega/Inputs/Digital Processor/Reverse Activation/Enabled Subsystem ==
  Enable : EnablePort  StatesWhenEnabling=reset
  Add : Sum
  Constant : Constant  Value=0.1
  Unit Delay : UnitDelay  SampleTime=-1  HasFrameUpgradeWarning=on
  Out1 : Outport
  wires:
  Unit Delay/1 -> Add/2
  Constant/1 -> Add/1
  Add/1 -> Unit Delay/1, Out1/1

== system eBike_simulink_arduinoMega/Inputs/Digital Processor/Wake/Enabled Subsystem ==
  Enable : EnablePort  StatesWhenEnabling=reset
  Add : Sum
  Constant : Constant  Value=0.1
  Unit Delay : UnitDelay  SampleTime=-1  HasFrameUpgradeWarning=on
  Out1 : Outport
  wires:
  Unit Delay/1 -> Add/2
  Constant/1 -> Add/1
  Add/1 -> Unit Delay/1, Out1/1

== system eBike_simulink_arduinoMega/Inputs/Digital Processor/Wake/Subsystem ==
  Set : Inport
  Reset : Inport  Port=2
  Constant2 : Constant
  Constant3 : Constant  Value=0
  Multiport Switch3 : MultiPortSwitch  DataPortOrder=Zero-based contiguous  Inputs=2  zeroidx=on
  Multiport Switch4 : MultiPortSwitch  DataPortOrder=Zero-based contiguous  Inputs=2  zeroidx=on
  Unit Delay1 : UnitDelay  SampleTime=-1  HasFrameUpgradeWarning=on
  Out1 : Outport
  wires:
  Set/1 -> Multiport Switch3/1
  Constant2/1 -> Multiport Switch3/3
  Multiport Switch3/1 -> Multiport Switch4/2
  Unit Delay1/1 -> Multiport Switch3/2
  Multiport Switch4/1 -> Out1/1, Unit Delay1/1
  Constant3/1 -> Multiport Switch4/3
  Reset/1 -> Multiport Switch4/1

== stateflow chart eBike_simulink_arduinoMega/Control/Mode LED/Chart ==
  state MCU_Off
    relay_LED = Startup_LED
  state MCU_On
    state Startup
      relay_LED = Startup_LED
    state Pedal_Asisst
      entry:
      tmr_p = 0;
      during:
      tmr_p = tmr_p + 1;
    state Cruise_Control
      entry:
      tmr_c = 0;
      during:
      tmr_c = tmr_c + 1;
    state Reverse
      entry:
      tmr_r = 0;
      during:
      tmr_r = tmr_r + 1;
    state Reverse_Off
      entry:
      relay_LED = boolean(1);
      tmr_ro = 0;
      during:
      tmr_ro = tmr_ro + 1;
    (default) -> Startup
    Startup -> Pedal_Asisst [order 1] : [PA_LED==1]{relay_LED = boolean(1)}
    Pedal_Asisst -> Pedal_Asisst [order 2] : [tmr_p > 50]{relay_LED = ~(relay_LED)}
    Pedal_Asisst -> Startup [order 1] : [PA_LED==0]
    Cruise_Control -> Startup [order 1] : [CC_LED==0]
    Startup -> Cruise_Control [order 2] : [CC_LED==1]{relay_LED = boolean(1)}
    Reverse -> Startup [order 1] : [Rev_LED==0]
    Startup -> Reverse [order 3] : [Rev_LED==1]{relay_LED = boolean(1)}
    Reverse -> Reverse [order 2] : [tmr_r>15]{relay_LED=~(relay_LED),cnt=cnt+1}
    Cruise_Control -> Cruise_Control [order 2] : [tmr_c>20]{relay_LED=~(relay_LED)}
    Reverse_Off -> Reverse : [tmr_ro>50]
    Reverse -> Reverse_Off [order 3] : [cnt>=6]{cnt=0}
  (default) -> MCU_Off
  MCU_Off -> MCU_On : [MCU_Wake==0]
  MCU_On -> MCU_Off : [MCU_Wake==1]
  data: MCU_Wake input; Startup_LED input; CC_LED input; Rev_LED input; PA_LED input; relay_LED output boolean; tmr_p local; tmr_c local; tmr_r local; cnt local =0; tmr_ro local

== stateflow chart eBike_simulink_arduinoMega/Control/Startup/Chart ==
  state Driver
    state Diagnostic_On
      entry:
      ssr_control = 0
      relay_led = 0;
      tmr_d = 0;
      during:
      tmr_d = tmr_d + 1;
      exit:
      relay_led = 1;
    state Buffer_Mode
      entry:
      ssr_control = 1;
      mcu_wake =1;
      tmr_b = 0;
      during:
      tmr_b = tmr_b + 1;
      exit:
      tmr_b  = 0;
    state MCU_Drive
      state Throttle_Enable
        throttle_vld = 1;
        exit:
        throttle_vld=0;
      state MCU_init
        entry:
        mcu_wake = 0;
        relay_led = 0;
      (default) -> MCU_init
      MCU_init -> Throttle_Enable : [Th_Po>4&&Th_Po<6]
      Throttle_Enable -> MCU_init : [~(Th_Po>4&&Th_Po<6)]
    (default) -> Diagnostic_On
    Diagnostic_On -> Buffer_Mode [order 1] : [tmr_d>=20&&Ba_Cu==0&&Ba_V>=30]{tmr_d=0}
    Buffer_Mode -> Diagnostic_On [order 1] : [tmr_b > 300]
    Buffer_Mode -> (junction 52) [order 2] : [Mode==1&&tmr_b>=20]
    (junction 52) -> Buffer_Mode [order 2]
    Buffer_Mode -> (junction 52) [order 3] : [Cu_Wa==1&&tmr_b>=20]{Cu_Wa=0}
    (junction 52) -> MCU_Drive [order 1] : [Th_Per<=10&&Ba_Cu<12&&cnt<=5&&MCU_Wake==1]
    MCU_Drive -> Buffer_Mode [order 2] : [Ba_V<30]{cnt = cnt + 1}
    MCU_Drive -> Buffer_Mode [order 1] : [Ba_Cu>12]{Cu_Wa=1}
  state Init
    entry:
    throttle_vld = 0;
    relay_led = 1;
    mcu_wake = 1;
    ssr_control = 0;
    cnt = 0;
  (default) -> Init
  Driver -> Init : [Ba_Cu>15]{Fault=1}
  Diagnostic_On -> Init [order 2] : [tmr_d > 18&&cnt>5]{Fault=1}
  Init -> Diagnostic_On : [Fault==0]
  data: mcu_wake output; throttle_vld output; ssr_control output; relay_led output; Ba_Cu input; MCU_Wake input; Th_Per input; Mode input; Ba_V input; Fault local =0; Th_Po input; Cu_Wa local; cnt output; tmr_b output; tmr_d output
